simulink model "test"  (R2022a)
settings: Solver=FixedStepAuto  StartTime=0.0  StopTime=50  FixedStep=0.01  RelTol=1e-3
model workspace (MAT data in the model file):
  slope = 30
libraries: slpidlib x1
settings Model: Creator=黃冠融  LastModifiedBy=黃冠融

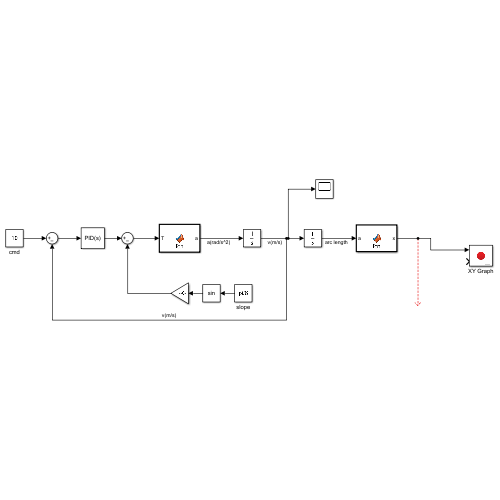
[thumbnail: Simulink's stored preview of the top-level diagram]
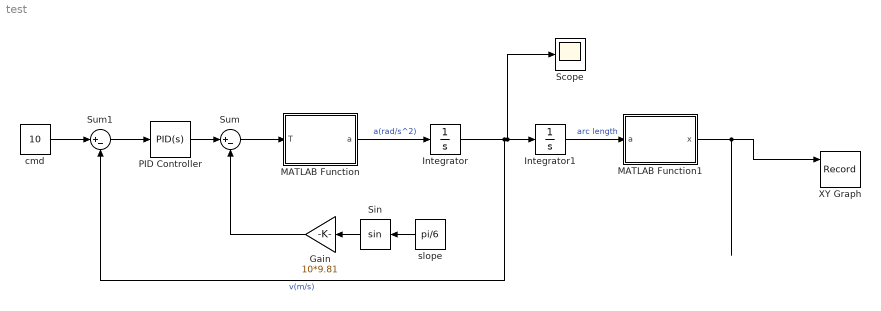
== system test ==
  Gain : Gain  Gain=10*9.81
  Integrator : Integrator
  Integrator1 : Integrator
  MATLAB Function : MATLAB Function  TreatAsAtomicUnit=on
  MATLAB Function1 : MATLAB Function  TreatAsAtomicUnit=on
  PID Controller : slpidlib/PID Controller  Controller=PID  Form=Parallel  TimeDomain=Continuous-time  UseExternalTs=off  SampleTime=-1  IntegratorMethod=Forward Euler  FilterMethod=Forward Euler  ControllerParametersSource=internal  P=1  I=1  UseKiTs=off  D=0  N=100  UseFilter=on  TunerSelectOption=Transfer Function Based (PID Tuner App)  InitialConditionSource=internal  InitialConditionForIntegrator=0  InitialConditionForFilter=0  DifferentiatorICPrevScaledInput=0  ExternalReset=none  TrackingMode=off  Kt=1  LimitOutput=off  SatLimitsSource=internal  UpperSaturationLimit=inf  LowerSaturationLimit=-inf  LinearizeAsGain=on  AntiWindupMode=none  Kb=1  POutMin=[]  POutMax=[]  IOutMin=[]  IOutMax=[]  DOutMin=[]  DOutMax=[]  NOutMin=[]  NOutMax=[]  SumOutMin=[]  SumOutMax=[]  SaturationOutMin=[]  SaturationOutMax=[]  PParamMin=[]  PParamMax=[]  IParamMin=[]  IParamMax=[]  DParamMin=[]  DParamMax=[]  NParamMin=[]  NParamMax=[]  KbParamMin=[]  KbParamMax=[]  KtParamMin=[]  KtParamMax=[]  KbOutMin=[]  KbOutMax=[]  KtOutMin=[]  KtOutMax=[]  IntegratorOutMin=[]  IntegratorOutMax=[]  FilterOutMin=[]  FilterOutMax=[]  SumI1OutMin=[]  SumI1OutMax=[]  SumI2OutMin=[]  SumI2OutMax=[]  SumI3OutMin=[]  SumI3OutMax=[]  SumI4OutMin=[]  SumI4OutMax=[]  SumDOutMin=[]  SumDOutMax=[]  DifferentiatorOutMin=[]  DifferentiatorOutMax=[]  FilterDiffOutCoefMin=[]  FilterDiffOutCoefMax=[]  ReciprocalOutMin=[]  ReciprocalOutMax=[]  SumDenOutMin=[]  SumDenOutMax=[]  SumNumOutMin=[]  SumNumOutMax=[]  DivideOutMin=[]  DivideOutMax=[]  UdiffTsProdOutMin=[]  UdiffTsProdOutMax=[]  NTsProdOutMin=[]  NTsProdOutMax=[]  UintegralTsProdOutMin=[]  UintegralTsProdOutMax=[]  UngainTsProdOutMin=[]  UngainTsProdOutMax=[]  IntegratorContinuousStateAttributes=''  IntegratorStateMustResolveToSignalObject=off  IntegratorRTWStateStorageClass=Auto  FilterContinuousStateAttributes=''  FilterStateMustResolveToSignalObject=off  FilterRTWStateStorageClass=Auto  ParallelPVariant=InternalParameters  IdealPVariant=Disabled  IVariant=InternalParameters  DVariant=InternalParameters  IntegratorVariant=Continuous  SatVariant=Disabled  AWVariant=Passthrough  PCopyVariant=Disabled  TRVariant=Disabled  FdbkBlocksVariant=Forward  IdealPFdbkVariant=Disabled  SatFdbkVariant=Disabled  DerivativeFilterVariant=ContFilter  NVariant=InternalParameters  NCopyVariant=Disabled  FilterICVariant=InternalICsFilter  IntegratorICVariant=InternalICs  ExternalResetVariant=Disabled  TRSumVariant=Passthrough  SumFdbkVariant=Disabled  SumVariant=Sum_PID  TsampFilterVariant=InternalTs  TsampNgainVariant=Passthrough  TsampIntegralVariant=Passthrough  ExternalSaturationOutDataTypeStr=Inherit: Same as second input  aMode=0
  Scope : Scope
  Sin : Trigonometry
  Sum : Sum  Inputs=|+-
  Sum1 : Sum  Inputs=|+-
  XY Graph : Record  FileSettingsInternal="{\"entries\":[{\"content\":{\"excelSettings\":{\"content\":{},\"type\":\"Streamout.ExcelSettings\"}},\"type\":\"Streamout.FileSettingStorage\",\"uuid\":\"421db442-906f-4df5-ae45-2d36c41a124b\"}],\"packageUris\":[\"http://schema.mathworks.com/mf0/streamout_blocks/R2020a\"],\"version\":\"1.0\"}"  Layout=[1 1]  SignalsInternal="{\"entries\":[{\"content\":{\"signals\":[{\"content\":{\"blockPath\":[\"test/XY Graph\"],\"channel\":[],\"dimensions\":[1],\"domain\":\"test/XY Graph\",\"lineColor\":\"#a2142f\",\"plots\":[1],\"port\":1,\"sid\":[\"\"],\"signalID\":20,\"signalName\":\"x\"},\"type\":\"RecordBlkView.Signal\",\"uuid\":\"f9dddc7a-656f-4761-aa9b-075bf58003b4\"},{\"content\":{\"blockPath\":[\"test/XY Graph\"],\"channel\":[],\"dimensions\":[1],\"domain\":\"test/XY Graph\",\"lineColor\":\"#139fff\",\"plots\":[1],\"port\":2,\"sid\":[\"\"],\"signalID\":24,\"signalName\":\"y\"},\"type\":\"RecordBlkView.Signal\",\"uuid\":\"9d527ee2-320f-4675-8a6f-4ee287dc2a93\"}]},\"type\":\"RecordBlkView.InputSignals\",\"uuid\":\"1aef8eef-0aef-497d-8205-d5f15d821430\"}],\"packageUris\":[\"http://schema.mathworks.com/mf0/streamout_blocks/R2020a\"],\"version\":\"1.0\"}"  VisualizationBindings="{\"xyplotplugin\":{\"info\":[{\"series\":[{\"bindingParametersList\":[{\"parameter\":\"X-Axis\",\"signalID\":20,\"signalName\":\"x\"},{\"parameter\":\"Y-Axis\",\"signalID\":24,\"signalName\":\"y\"}],\"seriesID\":25519}],\"subplotID\":1}]}}"  CompatibilityTag=XY
  cmd : Constant  Value=10
  slope : Constant  Value=pi/6
  wires:
  MATLAB Function/1(a) -> Integrator/1  "a(rad/s^2)"
  Integrator/1 -> Sum1/2, Scope/1, Integrator1/1  "v(m/s)"
  PID Controller/1 -> Sum/1
  Sum/1 -> MATLAB Function/1(T)
  Sin/1 -> Gain/1
  cmd/1 -> Sum1/1
  Sum1/1 -> PID Controller/1
  Gain/1 -> Sum/2
  slope/1 -> Sin/1
  Integrator1/1 -> MATLAB Function1/1(a)  "arc length"
  MATLAB Function1/1(x) -> XY Graph/1

== matlab function test/MATLAB Function ==
  data: T input; a output
function a= fcn(T)
I=10*2/5;
a=T/I;

== matlab function test/MATLAB Function1 ==
  data: a input; x output
function x = fcn(a)
x=(2^(1/6)*(2*2^(2/3) + ((9*a^2 - 32)^(1/2) - 3*a)^(2/3)))/((9*a^2 - 32)^(1/2) - 3*a)^(1/3)
